simulink model "x11"  (Simulink 7.2)
settings: Solver=ode45  StartTime=0.0  StopTime=10.0  RelTol=1e-3
libraries: cdsEpicsOut x289, cdsTP x288, cdsFilt x2, dac x2, cdsContec1616DIO x1, cdsParameters x1
(part 1 of 6)
settings Model: Creator=rolf  LastModifiedBy=rolf  ExtModeAutoUpdateStatusClock=off
settings OptimizationCC: InitFltsAndDblsToZero=on
settings DebuggingCC: SaveWithParameterizedLinksMsg=none  SignalResolutionControl=TryResolveAllWithWarning
settings GRTTargetCC: TargetFcnLib=ansi_tfl_tmw.mat

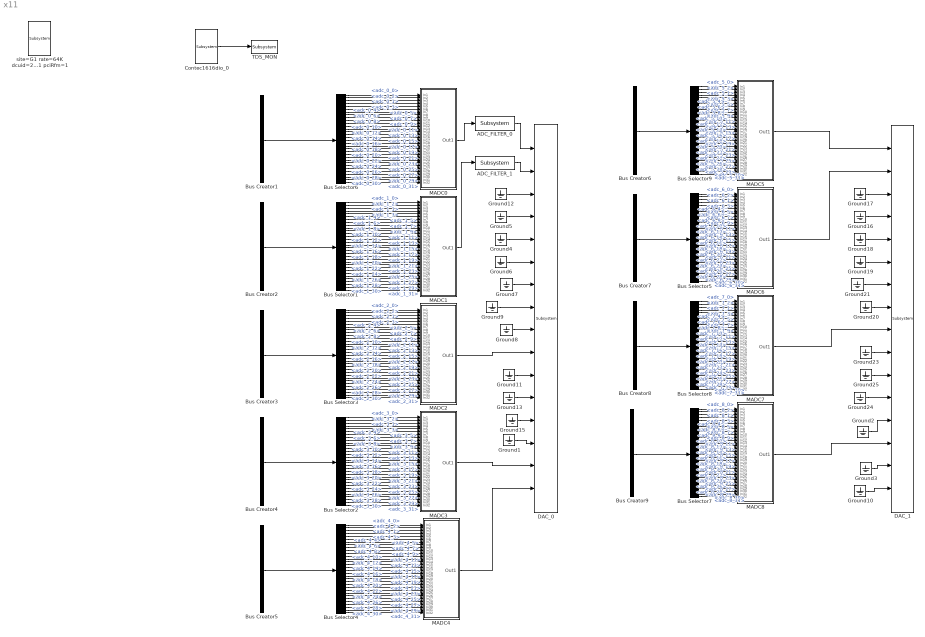
== system x11 ==
  ADC_FILTER_0 : cdsFilt/Subsystem  Tag=cdsFilt  Description=|  SystemSampleTime=-1
      | Purpose:                                                                                                                                                                                                                                  
      | Standard CDS IIR filter module.                                                                                                                                                                                                           
      |                                                                                                                                                                                                                                           
      | Operation:                                                                                                                                                                                                                                
      | Consists of 10 second order section IIR filters, plus a ramped gain stage. In FE code, also provides pre-defined test points and excitation channel inputs. The filter coefficients are defined in the LIGO system using the 'foton' tool.
      |                                                                                                                                                                                                                                           
      | Usage:                                                                                                                                                                                                                                    
      | Name the part with the desired filter module name.
      settings: AttributesFormatString=%<Tag>
  ADC_FILTER_1 : cdsFilt/Subsystem  Tag=cdsFilt  Description=|  SystemSampleTime=-1
      | Purpose:                                                                                                                                                                                                                                  
      | Standard CDS IIR filter module.                                                                                                                                                                                                           
      |                                                                                                                                                                                                                                           
      | Operation:                                                                                                                                                                                                                                
      | Consists of 10 second order section IIR filters, plus a ramped gain stage. In FE code, also provides pre-defined test points and excitation channel inputs. The filter coefficients are defined in the LIGO system using the 'foton' tool.
      |                                                                                                                                                                                                                                           
      | Usage:                                                                                                                                                                                                                                    
      | Name the part with the desired filter module name.
      settings: AttributesFormatString=%<Tag>
  Bus Creator1 : BusCreator  Tag=adc_0  Description=|  Inputs='adc_0_0','adc_0_1','adc_0_2','adc_0_3','adc_0_4','adc_0_5','adc_0_6','adc_0_7','adc_0_8','adc_0_9','adc_0_10','adc_0_11','adc_0_12','adc_0_13','adc_0_14','adc_0_15','adc_0_16','adc_0_17','adc_0_18','adc_0_19','adc_0_20','adc_0_21','adc_0_22','adc_0_23','adc_0_24','adc_0_25','adc_0_26','adc_0_27','adc_0_28','adc_0_29','adc_0_30','adc_0_31'
      | ADC0      
      | card_num=0
      settings: AttributesFormatString=%<Description>
  Bus Creator2 : BusCreator  Description=|  Inputs='adc_1_0','adc_1_1','adc_1_2','adc_1_3','adc_1_4','adc_1_5','adc_1_6','adc_1_7','adc_1_8','adc_1_9','adc_1_10','adc_1_11','adc_1_12','adc_1_13','adc_1_14','adc_1_15','adc_1_16','adc_1_17','adc_1_18','adc_1_19','adc_1_20','adc_1_21','adc_1_22','adc_1_23','adc_1_24','adc_1_25','adc_1_26','adc_1_27','adc_1_28','adc_1_29','adc_1_30','adc_1_31'
      | ADC1      
      | card_num=1
      settings: AttributesFormatString=%<Description>
  Bus Creator3 : BusCreator  Description=|  Inputs='adc_2_0','adc_2_1','adc_2_2','adc_2_3','adc_2_4','adc_2_5','adc_2_6','adc_2_7','adc_2_8','adc_2_9','adc_2_10','adc_2_11','adc_2_12','adc_2_13','adc_2_14','adc_2_15','adc_2_16','adc_2_17','adc_2_18','adc_2_19','adc_2_20','adc_2_21','adc_2_22','adc_2_23','adc_2_24','adc_2_25','adc_2_26','adc_2_27','adc_2_28','adc_2_29','adc_2_30','adc_2_31'
      | ADC2      
      | card_num=2
      settings: AttributesFormatString=%<Description>
  Bus Creator4 : BusCreator  Description=|  Inputs='adc_3_0','adc_3_1','adc_3_2','adc_3_3','adc_3_4','adc_3_5','adc_3_6','adc_3_7','adc_3_8','adc_3_9','adc_3_10','adc_3_11','adc_3_12','adc_3_13','adc_3_14','adc_3_15','adc_3_16','adc_3_17','adc_3_18','adc_3_19','adc_3_20','adc_3_21','adc_3_22','adc_3_23','adc_3_24','adc_3_25','adc_3_26','adc_3_27','adc_3_28','adc_3_29','adc_3_30','adc_3_31'
      | ADC3      
      | card_num=3
      settings: AttributesFormatString=%<Description>
  Bus Creator5 : BusCreator  Description=|  Inputs='adc_4_0','adc_4_1','adc_4_2','adc_4_3','adc_4_4','adc_4_5','adc_4_6','adc_4_7','adc_4_8','adc_4_9','adc_4_10','adc_4_11','adc_4_12','adc_4_13','adc_4_14','adc_4_15','adc_4_16','adc_4_17','adc_4_18','adc_4_19','adc_4_20','adc_4_21','adc_4_22','adc_4_23','adc_4_24','adc_4_25','adc_4_26','adc_4_27','adc_4_28','adc_4_29','adc_4_30','adc_4_31'
      | ADC4      
      | card_num=4
      settings: AttributesFormatString=%<Description>
  Bus Creator6 : BusCreator  Description=|  Inputs='adc_5_0','adc_5_1','adc_5_2','adc_5_3','adc_5_4','adc_5_5','adc_5_6','adc_5_7','adc_5_8','adc_5_9','adc_5_10','adc_5_11','adc_5_12','adc_5_13','adc_5_14','adc_5_15','adc_5_16','adc_5_17','adc_5_18','adc_5_19','adc_5_20','adc_5_21','adc_5_22','adc_5_23','adc_5_24','adc_5_25','adc_5_26','adc_5_27','adc_5_28','adc_5_29','adc_5_30','adc_5_31'
      | ADC5      
      | card_num=5
      settings: AttributesFormatString=%<Description>
  Bus Creator7 : BusCreator  Description=|  Inputs='adc_6_0','adc_6_1','adc_6_2','adc_6_3','adc_6_4','adc_6_5','adc_6_6','adc_6_7','adc_6_8','adc_6_9','adc_6_10','adc_6_11','adc_6_12','adc_6_13','adc_6_14','adc_6_15','adc_6_16','adc_6_17','adc_6_18','adc_6_19','adc_6_20','adc_6_21','adc_6_22','adc_6_23','adc_6_24','adc_6_25','adc_6_26','adc_6_27','adc_6_28','adc_6_29','adc_6_30','adc_6_31'
      | ADC6      
      | card_num=6
      settings: AttributesFormatString=%<Description>
  Bus Creator8 : BusCreator  Description=|  Inputs='adc_7_0','adc_7_1','adc_7_2','adc_7_3','adc_7_4','adc_7_5','adc_7_6','adc_7_7','adc_7_8','adc_7_9','adc_7_10','adc_7_11','adc_7_12','adc_7_13','adc_7_14','adc_7_15','adc_7_16','adc_7_17','adc_7_18','adc_7_19','adc_7_20','adc_7_21','adc_7_22','adc_7_23','adc_7_24','adc_7_25','adc_7_26','adc_7_27','adc_7_28','adc_7_29','adc_7_30','adc_7_31'
      | ADC7      
      | card_num=7
      settings: AttributesFormatString=%<Description>
  Bus Creator9 : BusCreator  Description=|  Inputs='adc_8_0','adc_8_1','adc_8_2','adc_8_3','adc_8_4','adc_8_5','adc_8_6','adc_8_7','adc_8_8','adc_8_9','adc_8_10','adc_8_11','adc_8_12','adc_8_13','adc_8_14','adc_8_15','adc_8_16','adc_8_17','adc_8_18','adc_8_19','adc_8_20','adc_8_21','adc_8_22','adc_8_23','adc_8_24','adc_8_25','adc_8_26','adc_8_27','adc_8_28','adc_8_29','adc_8_30','adc_8_31'
      | ADC8      
      | card_num=8
      settings: AttributesFormatString=%<Description>
  Bus Selector1 : BusSelector  Description=ADC Selector  OutputSignals=adc_1_0,adc_1_1,adc_1_2,adc_1_3,adc_1_4,adc_1_5,adc_1_6,adc_1_7,adc_1_8,adc_1_9,adc_1_10,adc_1_11,adc_1_12,adc_1_13,adc_1_14,adc_1_15,adc_1_16,adc_1_17,adc_1_18,adc_1_19,adc_1_20,adc_1_21,adc_1_22,adc_1_23,adc_1_24,adc_1_25,adc_1_26,adc_1_27,adc_1_28,adc_1_29,adc_1_30,adc_1_31
      settings: AttributesFormatString=%<Description>
  Bus Selector2 : BusSelector  Description=ADC Selector  OutputSignals=adc_3_0,adc_3_1,adc_3_2,adc_3_3,adc_3_4,adc_3_5,adc_3_6,adc_3_7,adc_3_8,adc_3_9,adc_3_10,adc_3_11,adc_3_12,adc_3_13,adc_3_14,adc_3_15,adc_3_16,adc_3_17,adc_3_18,adc_3_19,adc_3_20,adc_3_21,adc_3_22,adc_3_23,adc_3_24,adc_3_25,adc_3_26,adc_3_27,adc_3_28,adc_3_29,adc_3_30,adc_3_31
      settings: AttributesFormatString=%<Description>
  Bus Selector3 : BusSelector  Description=ADC Selector  OutputSignals=adc_2_0,adc_2_1,adc_2_2,adc_2_3,adc_2_4,adc_2_5,adc_2_6,adc_2_7,adc_2_8,adc_2_9,adc_2_10,adc_2_11,adc_2_12,adc_2_13,adc_2_14,adc_2_15,adc_2_16,adc_2_17,adc_2_18,adc_2_19,adc_2_20,adc_2_21,adc_2_22,adc_2_23,adc_2_24,adc_2_25,adc_2_26,adc_2_27,adc_2_28,adc_2_29,adc_2_30,adc_2_31
      settings: AttributesFormatString=%<Description>
  Bus Selector4 : BusSelector  Description=ADC Selector  OutputSignals=adc_4_0,adc_4_1,adc_4_2,adc_4_3,adc_4_4,adc_4_5,adc_4_6,adc_4_7,adc_4_8,adc_4_9,adc_4_10,adc_4_11,adc_4_12,adc_4_13,adc_4_14,adc_4_15,adc_4_16,adc_4_17,adc_4_18,adc_4_19,adc_4_20,adc_4_21,adc_4_22,adc_4_23,adc_4_24,adc_4_25,adc_4_26,adc_4_27,adc_4_28,adc_4_29,adc_4_30,adc_4_31
      settings: AttributesFormatString=%<Description>
  Bus Selector5 : BusSelector  Description=ADC Selector  OutputSignals=adc_6_0,adc_6_1,adc_6_2,adc_6_3,adc_6_4,adc_6_5,adc_6_6,adc_6_7,adc_6_8,adc_6_9,adc_6_10,adc_6_11,adc_6_12,adc_6_13,adc_6_14,adc_6_15,adc_6_16,adc_6_17,adc_6_18,adc_6_19,adc_6_20,adc_6_21,adc_6_22,adc_6_23,adc_6_24,adc_6_25,adc_6_26,adc_6_27,adc_6_28,adc_6_29,adc_6_30,adc_6_31
      settings: AttributesFormatString=%<Description>
  Bus Selector6 : BusSelector  Description=ADC Selector  OutputSignals=adc_0_0,adc_0_1,adc_0_2,adc_0_3,adc_0_4,adc_0_5,adc_0_6,adc_0_7,adc_0_8,adc_0_9,adc_0_10,adc_0_11,adc_0_12,adc_0_13,adc_0_14,adc_0_15,adc_0_16,adc_0_17,adc_0_18,adc_0_19,adc_0_20,adc_0_21,adc_0_22,adc_0_23,adc_0_24,adc_0_25,adc_0_26,adc_0_27,adc_0_28,adc_0_29,adc_0_30,adc_0_31
      settings: AttributesFormatString=%<Description>
  Bus Selector7 : BusSelector  Description=ADC Selector  OutputSignals=adc_8_0,adc_8_1,adc_8_2,adc_8_3,adc_8_4,adc_8_5,adc_8_6,adc_8_7,adc_8_8,adc_8_9,adc_8_10,adc_8_11,adc_8_12,adc_8_13,adc_8_14,adc_8_15,adc_8_16,adc_8_17,adc_8_18,adc_8_19,adc_8_20,adc_8_21,adc_8_22,adc_8_23,adc_8_24,adc_8_25,adc_8_26,adc_8_27,adc_8_28,adc_8_29,adc_8_30,adc_8_31
      settings: AttributesFormatString=%<Description>
  Bus Selector8 : BusSelector  Description=ADC Selector  OutputSignals=adc_7_0,adc_7_1,adc_7_2,adc_7_3,adc_7_4,adc_7_5,adc_7_6,adc_7_7,adc_7_8,adc_7_9,adc_7_10,adc_7_11,adc_7_12,adc_7_13,adc_7_14,adc_7_15,adc_7_16,adc_7_17,adc_7_18,adc_7_19,adc_7_20,adc_7_21,adc_7_22,adc_7_23,adc_7_24,adc_7_25,adc_7_26,adc_7_27,adc_7_28,adc_7_29,adc_7_30,adc_7_31
      settings: AttributesFormatString=%<Description>
  Bus Selector9 : BusSelector  Description=ADC Selector  OutputSignals=adc_5_0,adc_5_1,adc_5_2,adc_5_3,adc_5_4,adc_5_5,adc_5_6,adc_5_7,adc_5_8,adc_5_9,adc_5_10,adc_5_11,adc_5_12,adc_5_13,adc_5_14,adc_5_15,adc_5_16,adc_5_17,adc_5_18,adc_5_19,adc_5_20,adc_5_21,adc_5_22,adc_5_23,adc_5_24,adc_5_25,adc_5_26,adc_5_27,adc_5_28,adc_5_29,adc_5_30,adc_5_31
      settings: AttributesFormatString=%<Description>
  Contec1616dio_0 : cdsContec1616DIO/Subsystem  Tag=cdsCDIO1616  SystemSampleTime=-1
      settings: AttributesFormatString=%<Tag>
  DAC_0 : dac/Subsystem  Description=card_num=0  SystemSampleTime=-1
  DAC_1 : dac/Subsystem  Description=card_num=1  SystemSampleTime=-1
  Ground{1..13,15..21,23..25} (23 alike) : Ground
  MADC0 : Subsystem
  MADC1 : Subsystem
  MADC2 : Subsystem
  MADC3 : Subsystem
  MADC4 : Subsystem
  MADC5 : Subsystem
  MADC6 : Subsystem
  MADC7 : Subsystem
  MADC8 : Subsystem
  TDS_MON : cdsEpicsOut/Subsystem  Tag=cdsEpicsOutput  Description=|  SystemSampleTime=-1
      | Purpose:                                          
      | Output a FE signal to an EPICS channel.           
      |                                                   
      | Operation:                                        
      | Takes input value and passes it to EPICS record.  
      |                                                   
      | Usage:                                            
      | Name the part with the desired EPICS rrecord name.
      settings: AttributesFormatString=%<Tag>
  site=G1 rate=64K dcuid=25 shmem_daq=1 gds_node_id=6 adcMaster=1 pciRfm=1 : cdsParameters/Subsystem  Tag=cdsParameters  SystemSampleTime=-1
      settings: AttributesFormatString=%<Tag>
  wires:
  Ground15/1 -> DAC_0/13
  Ground1/1 -> DAC_0/14
  Bus Creator1/1 -> Bus Selector6/1
  Ground5/1 -> DAC_0/4
  Ground4/1 -> DAC_0/5
  Ground6/1 -> DAC_0/6
  Ground7/1 -> DAC_0/7
  Ground9/1 -> DAC_0/8
  Ground8/1 -> DAC_0/9
  Ground11/1 -> DAC_0/11
  Ground13/1 -> DAC_0/12
  Ground12/1 -> DAC_0/3
  Ground17/1 -> DAC_1/3
  Ground16/1 -> DAC_1/4
  Ground18/1 -> DAC_1/5
  Ground19/1 -> DAC_1/6
  Ground21/1 -> DAC_1/7
  Ground20/1 -> DAC_1/8
  Ground23/1 -> DAC_1/10
  Ground25/1 -> DAC_1/11
  Ground24/1 -> DAC_1/12
  Contec1616dio_0/1 -> TDS_MON/1
  Bus Creator2/1 -> Bus Selector1/1
  Bus Creator3/1 -> Bus Selector3/1
  Bus Creator4/1 -> Bus Selector2/1
  Bus Creator5/1 -> Bus Selector4/1
  Bus Creator6/1 -> Bus Selector9/1
  Bus Creator7/1 -> Bus Selector5/1
  Bus Creator8/1 -> Bus Selector8/1
  Ground2/1 -> DAC_1/13
  Ground3/1 -> DAC_1/15
  Ground10/1 -> DAC_1/16
  Bus Creator9/1 -> Bus Selector7/1
  MADC0/1(Out1) -> ADC_FILTER_0/1
  ADC_FILTER_0/1 -> DAC_0/1
  ADC_FILTER_1/1 -> DAC_0/2
  Bus Selector6/1 -> MADC0/1(In1)  "<adc_0_0>"
  Bus Selector6/2 -> MADC0/2(In2)  "<adc_0_1>"
  Bus Selector6/3 -> MADC0/3(In3)  "<adc_0_2>"
  Bus Selector6/4 -> MADC0/4(In4)  "<adc_0_3>"
  Bus Selector6/5 -> MADC0/5(In5)  "<adc_0_4>"
  Bus Selector6/6 -> MADC0/6(In6)  "<adc_0_5>"
  Bus Selector6/7 -> MADC0/7(In7)  "<adc_0_6>"
  Bus Selector6/8 -> MADC0/8(In8)  "<adc_0_7>"
  Bus Selector6/9 -> MADC0/9(In9)  "<adc_0_8>"
  Bus Selector6/10 -> MADC0/10(In10)  "<adc_0_9>"
  Bus Selector6/11 -> MADC0/11(In11)  "<adc_0_10>"
  Bus Selector6/12 -> MADC0/12(In12)  "<adc_0_11>"
  Bus Selector6/13 -> MADC0/13(In13)  "<adc_0_12>"
  Bus Selector6/14 -> MADC0/14(In14)  "<adc_0_13>"
  Bus Selector6/15 -> MADC0/15(In15)  "<adc_0_14>"
  Bus Selector6/16 -> MADC0/16(In16)  "<adc_0_15>"
  Bus Selector6/17 -> MADC0/17(In17)  "<adc_0_16>"
  Bus Selector6/18 -> MADC0/18(In18)  "<adc_0_17>"
  Bus Selector6/19 -> MADC0/19(In19)  "<adc_0_18>"
  Bus Selector6/20 -> MADC0/20(In20)  "<adc_0_19>"
  Bus Selector6/21 -> MADC0/21(In21)  "<adc_0_20>"
  Bus Selector6/22 -> MADC0/22(In22)  "<adc_0_21>"
  Bus Selector6/23 -> MADC0/23(In23)  "<adc_0_22>"
  Bus Selector6/24 -> MADC0/24(In24)  "<adc_0_23>"
  Bus Selector6/25 -> MADC0/25(In25)  "<adc_0_24>"
  Bus Selector6/26 -> MADC0/26(In26)  "<adc_0_25>"
  Bus Selector6/27 -> MADC0/27(In27)  "<adc_0_26>"
  Bus Selector6/28 -> MADC0/28(In28)  "<adc_0_27>"
  Bus Selector6/29 -> MADC0/29(In29)  "<adc_0_28>"
  Bus Selector6/30 -> MADC0/30(In30)  "<adc_0_29>"
  Bus Selector6/31 -> MADC0/31(In31)  "<adc_0_30>"
  Bus Selector6/32 -> MADC0/32(In32)  "<adc_0_31>"
  MADC3/1(Out1) -> DAC_0/15
  MADC4/1(Out1) -> DAC_0/16
  MADC2/1(Out1) -> DAC_0/10
  MADC1/1(Out1) -> ADC_FILTER_1/1
  MADC5/1(Out1) -> DAC_1/1
  MADC6/1(Out1) -> DAC_1/2
  MADC7/1(Out1) -> DAC_1/9
  MADC8/1(Out1) -> DAC_1/14
  Bus Selector1/1 -> MADC1/1(In1)  "<adc_1_0>"
  Bus Selector1/2 -> MADC1/2(In2)  "<adc_1_1>"
  Bus Selector1/3 -> MADC1/3(In3)  "<adc_1_2>"
  Bus Selector1/4 -> MADC1/4(In4)  "<adc_1_3>"
  Bus Selector1/5 -> MADC1/5(In5)  "<adc_1_4>"
  Bus Selector1/6 -> MADC1/6(In6)  "<adc_1_5>"
  Bus Selector1/7 -> MADC1/7(In7)  "<adc_1_6>"
  Bus Selector1/8 -> MADC1/8(In8)  "<adc_1_7>"
  Bus Selector1/9 -> MADC1/9(In9)  "<adc_1_8>"
  Bus Selector1/10 -> MADC1/10(In10)  "<adc_1_9>"
  Bus Selector1/11 -> MADC1/11(In11)  "<adc_1_10>"
  Bus Selector1/12 -> MADC1/12(In12)  "<adc_1_11>"
  Bus Selector1/13 -> MADC1/13(In13)  "<adc_1_12>"
  Bus Selector1/14 -> MADC1/14(In14)  "<adc_1_13>"
  Bus Selector1/15 -> MADC1/15(In15)  "<adc_1_14>"
  Bus Selector1/16 -> MADC1/16(In16)  "<adc_1_15>"
  Bus Selector1/17 -> MADC1/17(In17)  "<adc_1_16>"
  Bus Selector1/18 -> MADC1/18(In18)  "<adc_1_17>"
  Bus Selector1/19 -> MADC1/19(In19)  "<adc_1_18>"
  Bus Selector1/20 -> MADC1/20(In20)  "<adc_1_19>"
  Bus Selector1/21 -> MADC1/21(In21)  "<adc_1_20>"
  Bus Selector1/22 -> MADC1/22(In22)  "<adc_1_21>"
  Bus Selector1/23 -> MADC1/23(In23)  "<adc_1_22>"
  Bus Selector1/24 -> MADC1/24(In24)  "<adc_1_23>"
  Bus Selector1/25 -> MADC1/25(In25)  "<adc_1_24>"
  Bus Selector1/26 -> MADC1/26(In26)  "<adc_1_25>"
  Bus Selector1/27 -> MADC1/27(In27)  "<adc_1_26>"
  Bus Selector1/28 -> MADC1/28(In28)  "<adc_1_27>"
  Bus Selector1/29 -> MADC1/29(In29)  "<adc_1_28>"
  Bus Selector1/30 -> MADC1/30(In30)  "<adc_1_29>"
  Bus Selector1/31 -> MADC1/31(In31)  "<adc_1_30>"
  Bus Selector1/32 -> MADC1/32(In32)  "<adc_1_31>"
  Bus Selector3/1 -> MADC2/1(In1)  "<adc_2_0>"
  Bus Selector3/2 -> MADC2/2(In2)  "<adc_2_1>"
  Bus Selector3/3 -> MADC2/3(In3)  "<adc_2_2>"
  Bus Selector3/4 -> MADC2/4(In4)  "<adc_2_3>"
  Bus Selector3/5 -> MADC2/5(In5)  "<adc_2_4>"
  Bus Selector3/6 -> MADC2/6(In6)  "<adc_2_5>"
  Bus Selector3/7 -> MADC2/7(In7)  "<adc_2_6>"
  Bus Selector3/8 -> MADC2/8(In8)  "<adc_2_7>"
  Bus Selector3/9 -> MADC2/9(In9)  "<adc_2_8>"
  Bus Selector3/10 -> MADC2/10(In10)  "<adc_2_9>"
  Bus Selector3/11 -> MADC2/11(In11)  "<adc_2_10>"
  Bus Selector3/12 -> MADC2/12(In12)  "<adc_2_11>"
  Bus Selector3/13 -> MADC2/13(In13)  "<adc_2_12>"
  Bus Selector3/14 -> MADC2/14(In14)  "<adc_2_13>"
  Bus Selector3/15 -> MADC2/15(In15)  "<adc_2_14>"
  Bus Selector3/16 -> MADC2/16(In16)  "<adc_2_15>"
  Bus Selector3/17 -> MADC2/17(In17)  "<adc_2_16>"
  Bus Selector3/18 -> MADC2/18(In18)  "<adc_2_17>"
  Bus Selector3/19 -> MADC2/19(In19)  "<adc_2_18>"
  Bus Selector3/20 -> MADC2/20(In20)  "<adc_2_19>"
  Bus Selector3/21 -> MADC2/21(In21)  "<adc_2_20>"
  Bus Selector3/22 -> MADC2/22(In22)  "<adc_2_21>"
  Bus Selector3/23 -> MADC2/23(In23)  "<adc_2_22>"
  Bus Selector3/24 -> MADC2/24(In24)  "<adc_2_23>"
  Bus Selector3/25 -> MADC2/25(In25)  "<adc_2_24>"
  Bus Selector3/26 -> MADC2/26(In26)  "<adc_2_25>"
  Bus Selector3/27 -> MADC2/27(In27)  "<adc_2_26>"
  Bus Selector3/28 -> MADC2/28(In28)  "<adc_2_27>"
  Bus Selector3/29 -> MADC2/29(In29)  "<adc_2_28>"
  Bus Selector3/30 -> MADC2/30(In30)  "<adc_2_29>"
  Bus Selector3/31 -> MADC2/31(In31)  "<adc_2_30>"
  Bus Selector3/32 -> MADC2/32(In32)  "<adc_2_31>"
  Bus Selector2/1 -> MADC3/1(In1)  "<adc_3_0>"
  Bus Selector2/2 -> MADC3/2(In2)  "<adc_3_1>"
  Bus Selector2/3 -> MADC3/3(In3)  "<adc_3_2>"
  Bus Selector2/4 -> MADC3/4(In4)  "<adc_3_3>"
  Bus Selector2/5 -> MADC3/5(In5)  "<adc_3_4>"
  Bus Selector2/6 -> MADC3/6(In6)  "<adc_3_5>"
  Bus Selector2/7 -> MADC3/7(In7)  "<adc_3_6>"
  Bus Selector2/8 -> MADC3/8(In8)  "<adc_3_7>"
  Bus Selector2/9 -> MADC3/9(In9)  "<adc_3_8>"
  Bus Selector2/10 -> MADC3/10(In10)  "<adc_3_9>"
  Bus Selector2/11 -> MADC3/11(In11)  "<adc_3_10>"
  Bus Selector2/12 -> MADC3/12(In12)  "<adc_3_11>"
  Bus Selector2/13 -> MADC3/13(In13)  "<adc_3_12>"
  Bus Selector2/14 -> MADC3/14(In14)  "<adc_3_13>"
  Bus Selector2/15 -> MADC3/15(In15)  "<adc_3_14>"
  Bus Selector2/16 -> MADC3/16(In16)  "<adc_3_15>"
  Bus Selector2/17 -> MADC3/17(In17)  "<adc_3_16>"
  Bus Selector2/18 -> MADC3/18(In18)  "<adc_3_17>"
  Bus Selector2/19 -> MADC3/19(In19)  "<adc_3_18>"
  Bus Selector2/20 -> MADC3/20(In20)  "<adc_3_19>"
  Bus Selector2/21 -> MADC3/21(In21)  "<adc_3_20>"
  Bus Selector2/22 -> MADC3/22(In22)  "<adc_3_21>"
  Bus Selector2/23 -> MADC3/23(In23)  "<adc_3_22>"
  Bus Selector2/24 -> MADC3/24(In24)  "<adc_3_23>"
  Bus Selector2/25 -> MADC3/25(In25)  "<adc_3_24>"
  Bus Selector2/26 -> MADC3/26(In26)  "<adc_3_25>"
  Bus Selector2/27 -> MADC3/27(In27)  "<adc_3_26>"
  Bus Selector2/28 -> MADC3/28(In28)  "<adc_3_27>"
  Bus Selector2/29 -> MADC3/29(In29)  "<adc_3_28>"
  Bus Selector2/30 -> MADC3/30(In30)  "<adc_3_29>"
  Bus Selector2/31 -> MADC3/31(In31)  "<adc_3_30>"
  Bus Selector2/32 -> MADC3/32(In32)  "<adc_3_31>"
  Bus Selector4/1 -> MADC4/1(In1)  "<adc_4_0>"
  Bus Selector4/2 -> MADC4/2(In2)  "<adc_4_1>"
  Bus Selector4/3 -> MADC4/3(In3)  "<adc_4_2>"
  Bus Selector4/4 -> MADC4/4(In4)  "<adc_4_3>"
  Bus Selector4/5 -> MADC4/5(In5)  "<adc_4_4>"
  Bus Selector4/6 -> MADC4/6(In6)  "<adc_4_5>"
  Bus Selector4/7 -> MADC4/7(In7)  "<adc_4_6>"
  Bus Selector4/8 -> MADC4/8(In8)  "<adc_4_7>"
  Bus Selector4/9 -> MADC4/9(In9)  "<adc_4_8>"
  Bus Selector4/10 -> MADC4/10(In10)  "<adc_4_9>"
  Bus Selector4/11 -> MADC4/11(In11)  "<adc_4_10>"
  Bus Selector4/12 -> MADC4/12(In12)  "<adc_4_11>"
  Bus Selector4/13 -> MADC4/13(In13)  "<adc_4_12>"
  Bus Selector4/14 -> MADC4/14(In14)  "<adc_4_13>"
  Bus Selector4/15 -> MADC4/15(In15)  "<adc_4_14>"
  Bus Selector4/16 -> MADC4/16(In16)  "<adc_4_15>"
  Bus Selector4/17 -> MADC4/17(In17)  "<adc_4_16>"
  Bus Selector4/18 -> MADC4/18(In18)  "<adc_4_17>"
  Bus Selector4/19 -> MADC4/19(In19)  "<adc_4_18>"
  Bus Selector4/20 -> MADC4/20(In20)  "<adc_4_19>"
  Bus Selector4/21 -> MADC4/21(In21)  "<adc_4_20>"
  Bus Selector4/22 -> MADC4/22(In22)  "<adc_4_21>"
  Bus Selector4/23 -> MADC4/23(In23)  "<adc_4_22>"
  Bus Selector4/24 -> MADC4/24(In24)  "<adc_4_23>"
  Bus Selector4/25 -> MADC4/25(In25)  "<adc_4_24>"
  Bus Selector4/26 -> MADC4/26(In26)  "<adc_4_25>"
  Bus Selector4/27 -> MADC4/27(In27)  "<adc_4_26>"
  Bus Selector4/28 -> MADC4/28(In28)  "<adc_4_27>"
  Bus Selector4/29 -> MADC4/29(In29)  "<adc_4_28>"
  Bus Selector4/30 -> MADC4/30(In30)  "<adc_4_29>"
  Bus Selector4/31 -> MADC4/31(In31)  "<adc_4_30>"
  Bus Selector4/32 -> MADC4/32(In32)  "<adc_4_31>"
  Bus Selector9/1 -> MADC5/1(In1)  "<adc_5_0>"
  Bus Selector9/2 -> MADC5/2(In2)  "<adc_5_1>"
  Bus Selector9/3 -> MADC5/3(In3)  "<adc_5_2>"
  Bus Selector9/4 -> MADC5/4(In4)  "<adc_5_3>"
  Bus Selector9/5 -> MADC5/5(In5)  "<adc_5_4>"
  Bus Selector9/6 -> MADC5/6(In6)  "<adc_5_5>"
  Bus Selector9/7 -> MADC5/7(In7)  "<adc_5_6>"
  Bus Selector9/8 -> MADC5/8(In8)  "<adc_5_7>"
  Bus Selector9/9 -> MADC5/9(In9)  "<adc_5_8>"
  Bus Selector9/10 -> MADC5/10(In10)  "<adc_5_9>"
  Bus Selector9/11 -> MADC5/11(In11)  "<adc_5_10>"
  Bus Selector9/12 -> MADC5/12(In12)  "<adc_5_11>"
  Bus Selector9/13 -> MADC5/13(In13)  "<adc_5_12>"
  Bus Selector9/14 -> MADC5/14(In14)  "<adc_5_13>"
  Bus Selector9/15 -> MADC5/15(In15)  "<adc_5_14>"
  Bus Selector9/16 -> MADC5/16(In16)  "<adc_5_15>"
  Bus Selector9/17 -> MADC5/17(In17)  "<adc_5_16>"
  Bus Selector9/18 -> MADC5/18(In18)  "<adc_5_17>"
  Bus Selector9/19 -> MADC5/19(In19)  "<adc_5_18>"
  Bus Selector9/20 -> MADC5/20(In20)  "<adc_5_19>"
  Bus Selector9/21 -> MADC5/21(In21)  "<adc_5_20>"
  Bus Selector9/22 -> MADC5/22(In22)  "<adc_5_21>"
  Bus Selector9/23 -> MADC5/23(In23)  "<adc_5_22>"
  Bus Selector9/24 -> MADC5/24(In24)  "<adc_5_23>"
  Bus Selector9/25 -> MADC5/25(In25)  "<adc_5_24>"
  Bus Selector9/26 -> MADC5/26(In26)  "<adc_5_25>"
  Bus Selector9/27 -> MADC5/27(In27)  "<adc_5_26>"
  Bus Selector9/28 -> MADC5/28(In28)  "<adc_5_27>"
  Bus Selector9/29 -> MADC5/29(In29)  "<adc_5_28>"
  Bus Selector9/30 -> MADC5/30(In30)  "<adc_5_29>"
  Bus Selector9/31 -> MADC5/31(In31)  "<adc_5_30>"
  Bus Selector9/32 -> MADC5/32(In32)  "<adc_5_31>"
  Bus Selector5/1 -> MADC6/1(In1)  "<adc_6_0>"
  Bus Selector5/2 -> MADC6/2(In2)  "<adc_6_1>"
  Bus Selector5/3 -> MADC6/3(In3)  "<adc_6_2>"
  Bus Selector5/4 -> MADC6/4(In4)  "<adc_6_3>"
  Bus Selector5/5 -> MADC6/5(In5)  "<adc_6_4>"
  Bus Selector5/6 -> MADC6/6(In6)  "<adc_6_5>"
  Bus Selector5/7 -> MADC6/7(In7)  "<adc_6_6>"
  Bus Selector5/8 -> MADC6/8(In8)  "<adc_6_7>"
  Bus Selector5/9 -> MADC6/9(In9)  "<adc_6_8>"
  Bus Selector5/10 -> MADC6/10(In10)  "<adc_6_9>"
  Bus Selector5/11 -> MADC6/11(In11)  "<adc_6_10>"
  Bus Selector5/12 -> MADC6/12(In12)  "<adc_6_11>"
  Bus Selector5/13 -> MADC6/13(In13)  "<adc_6_12>"
  Bus Selector5/14 -> MADC6/14(In14)  "<adc_6_13>"
  Bus Selector5/15 -> MADC6/15(In15)  "<adc_6_14>"
  Bus Selector5/16 -> MADC6/16(In16)  "<adc_6_15>"
  Bus Selector5/17 -> MADC6/17(In17)  "<adc_6_16>"
  Bus Selector5/18 -> MADC6/18(In18)  "<adc_6_17>"
  Bus Selector5/19 -> MADC6/19(In19)  "<adc_6_18>"
  Bus Selector5/20 -> MADC6/20(In20)  "<adc_6_19>"
  Bus Selector5/21 -> MADC6/21(In21)  "<adc_6_20>"
  Bus Selector5/22 -> MADC6/22(In22)  "<adc_6_21>"
  Bus Selector5/23 -> MADC6/23(In23)  "<adc_6_22>"
  Bus Selector5/24 -> MADC6/24(In24)  "<adc_6_23>"
  Bus Selector5/25 -> MADC6/25(In25)  "<adc_6_24>"
  Bus Selector5/26 -> MADC6/26(In26)  "<adc_6_25>"
  Bus Selector5/27 -> MADC6/27(In27)  "<adc_6_26>"
  Bus Selector5/28 -> MADC6/28(In28)  "<adc_6_27>"
  Bus Selector5/29 -> MADC6/29(In29)  "<adc_6_28>"
  Bus Selector5/30 -> MADC6/30(In30)  "<adc_6_29>"
  Bus Selector5/31 -> MADC6/31(In31)  "<adc_6_30>"
  Bus Selector5/32 -> MADC6/32(In32)  "<adc_6_31>"
  Bus Selector8/1 -> MADC7/1(In1)  "<adc_7_0>"
  Bus Selector8/2 -> MADC7/2(In2)  "<adc_7_1>"
  Bus Selector8/3 -> MADC7/3(In3)  "<adc_7_2>"
  Bus Selector8/4 -> MADC7/4(In4)  "<adc_7_3>"
  Bus Selector8/5 -> MADC7/5(In5)  "<adc_7_4>"
  Bus Selector8/6 -> MADC7/6(In6)  "<adc_7_5>"
  Bus Selector8/7 -> MADC7/7(In7)  "<adc_7_6>"
  Bus Selector8/8 -> MADC7/8(In8)  "<adc_7_7>"
  Bus Selector8/9 -> MADC7/9(In9)  "<adc_7_8>"
  Bus Selector8/10 -> MADC7/10(In10)  "<adc_7_9>"
  Bus Selector8/11 -> MADC7/11(In11)  "<adc_7_10>"
  Bus Selector8/12 -> MADC7/12(In12)  "<adc_7_11>"
  Bus Selector8/13 -> MADC7/13(In13)  "<adc_7_12>"
  Bus Selector8/14 -> MADC7/14(In14)  "<adc_7_13>"
  Bus Selector8/15 -> MADC7/15(In15)  "<adc_7_14>"
  Bus Selector8/16 -> MADC7/16(In16)  "<adc_7_15>"
  Bus Selector8/17 -> MADC7/17(In17)  "<adc_7_16>"
  Bus Selector8/18 -> MADC7/18(In18)  "<adc_7_17>"
  Bus Selector8/19 -> MADC7/19(In19)  "<adc_7_18>"
  Bus Selector8/20 -> MADC7/20(In20)  "<adc_7_19>"
  Bus Selector8/21 -> MADC7/21(In21)  "<adc_7_20>"
  Bus Selector8/22 -> MADC7/22(In22)  "<adc_7_21>"
  Bus Selector8/23 -> MADC7/23(In23)  "<adc_7_22>"
  Bus Selector8/24 -> MADC7/24(In24)  "<adc_7_23>"
  Bus Selector8/25 -> MADC7/25(In25)  "<adc_7_24>"
  Bus Selector8/26 -> MADC7/26(In26)  "<adc_7_25>"
  Bus Selector8/27 -> MADC7/27(In27)  "<adc_7_26>"
  Bus Selector8/28 -> MADC7/28(In28)  "<adc_7_27>"
  Bus Selector8/29 -> MADC7/29(In29)  "<adc_7_28>"
  Bus Selector8/30 -> MADC7/30(In30)  "<adc_7_29>"
  Bus Selector8/31 -> MADC7/31(In31)  "<adc_7_30>"
  Bus Selector8/32 -> MADC7/32(In32)  "<adc_7_31>"
  Bus Selector7/1 -> MADC8/1(In1)  "<adc_8_0>"
  Bus Selector7/2 -> MADC8/2(In2)  "<adc_8_1>"
  Bus Selector7/3 -> MADC8/3(In3)  "<adc_8_2>"
  Bus Selector7/4 -> MADC8/4(In4)  "<adc_8_3>"
  Bus Selector7/5 -> MADC8/5(In5)  "<adc_8_4>"
  Bus Selector7/6 -> MADC8/6(In6)  "<adc_8_5>"
  Bus Selector7/7 -> MADC8/7(In7)  "<adc_8_6>"
  Bus Selector7/8 -> MADC8/8(In8)  "<adc_8_7>"
  Bus Selector7/9 -> MADC8/9(In9)  "<adc_8_8>"
  Bus Selector7/10 -> MADC8/10(In10)  "<adc_8_9>"
  Bus Selector7/11 -> MADC8/11(In11)  "<adc_8_10>"
  Bus Selector7/12 -> MADC8/12(In12)  "<adc_8_11>"
  Bus Selector7/13 -> MADC8/13(In13)  "<adc_8_12>"
  Bus Selector7/14 -> MADC8/14(In14)  "<adc_8_13>"
  Bus Selector7/15 -> MADC8/15(In15)  "<adc_8_14>"
  Bus Selector7/16 -> MADC8/16(In16)  "<adc_8_15>"
  Bus Selector7/17 -> MADC8/17(In17)  "<adc_8_16>"
  Bus Selector7/18 -> MADC8/18(In18)  "<adc_8_17>"
  Bus Selector7/19 -> MADC8/19(In19)  "<adc_8_18>"
  Bus Selector7/20 -> MADC8/20(In20)  "<adc_8_19>"
  Bus Selector7/21 -> MADC8/21(In21)  "<adc_8_20>"
  Bus Selector7/22 -> MADC8/22(In22)  "<adc_8_21>"
  Bus Selector7/23 -> MADC8/23(In23)  "<adc_8_22>"
  Bus Selector7/24 -> MADC8/24(In24)  "<adc_8_23>"
  Bus Selector7/25 -> MADC8/25(In25)  "<adc_8_24>"
  Bus Selector7/26 -> MADC8/26(In26)  "<adc_8_25>"
  Bus Selector7/27 -> MADC8/27(In27)  "<adc_8_26>"
  Bus Selector7/28 -> MADC8/28(In28)  "<adc_8_27>"
  Bus Selector7/29 -> MADC8/29(In29)  "<adc_8_28>"
  Bus Selector7/30 -> MADC8/30(In30)  "<adc_8_29>"
  Bus Selector7/31 -> MADC8/31(In31)  "<adc_8_30>"
  Bus Selector7/32 -> MADC8/32(In32)  "<adc_8_31>"
